simulink model "problem1Simulink"  (R2023a)
settings: Solver=VariableStepAuto  StartTime=0.0  StopTime=500  RelTol=1e-3
undefined symbols (not defined in the file): A, an, beta, Cd, Cr, g, m, rho, sgn, theta, Tm, wm
settings Model: Creator=qnmdgpqs  LastModifiedBy=qnmdgpqs

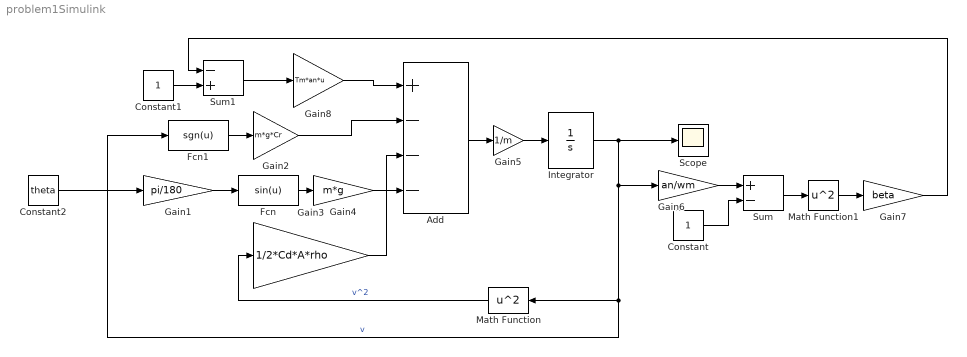
== system problem1Simulink ==
  Add : Sum  Inputs=+---
  Constant : Constant
  Constant1 : Constant
  Constant2 : Constant  Value=theta
  Fcn : Fcn  Expr=sin(u)
  Fcn1 : Fcn  Expr=sgn(u)
  Gain1 : Gain  Gain=pi/180
  Gain2 : Gain  Gain=m*g*Cr
  Gain3 : Gain  Gain=1/2*Cd*A*rho
  Gain4 : Gain  Gain=m*g
  Gain5 : Gain  Gain=1/m
  Gain6 : Gain  Gain=an/wm
  Gain7 : Gain  Gain=beta
  Gain8 : Gain  Gain=Tm*an*u
  Integrator : Integrator
  Math Function : Math  Operator=square
  Math Function1 : Math  Operator=square
  Scope : Scope
  Sum : Sum  Inputs=+-
  Sum1 : Sum  Inputs=-+
  wires:
  Math Function1/1 -> Gain7/1
  Constant1/1 -> Sum1/2
  Gain8/1 -> Add/1
  Math Function/1 -> Gain3/1  "v^2"
  Gain5/1 -> Integrator/1
  Gain2/1 -> Add/2
  Sum/1 -> Math Function1/1
  Gain4/1 -> Add/4
  Gain3/1 -> Add/3
  Add/1 -> Gain5/1
  Integrator/1 -> Fcn1/1, Math Function/1, Gain6/1, Scope/1  "v"
  Gain6/1 -> Sum/1
  Constant/1 -> Sum/2
  Gain7/1 -> Sum1/1
  Constant2/1 -> Gain1/1
  Fcn/1 -> Gain4/1
  Fcn1/1 -> Gain2/1
  Sum1/1 -> Gain8/1
  Gain1/1 -> Fcn/1
